simulink model "phase3_attitude_control"  (R2017b)
settings: Solver=VariableStepAuto  StartTime=0.0  StopTime=0.3  FixedStep=au  RelTol=1e-3
values from neighbouring files (symbols this model uses):
  c = 1.140*10^-7    (= 1.14e-07)    [Fcn_references_and_parameters.m]    (also in run_this_and_plot.m)
  Ix = 4.856*10^(-3)    (= 0.004856)    [Fcn_references_and_parameters.m]    (also in run_this_and_plot.m)
  Iy = 4.856*10^(-3)    (= 0.004856)    [Fcn_references_and_parameters.m]    (also in run_this_and_plot.m)
  Iz = 8.801*10^(-3)    (= 0.008801)    [Fcn_references_and_parameters.m]    (also in run_this_and_plot.m)
  k = 2.980*10^-6    (= 2.98e-06)    [Fcn_references_and_parameters.m]    (also in run_this_and_plot.m)
  l = 0.225    [Fcn_references_and_parameters.m]    (also in run_this_and_plot.m)
settings Model: Creator=Administrator  LastModifiedBy=chenjiasheng
settings CodeAppCC: StateflowObjectComments=on

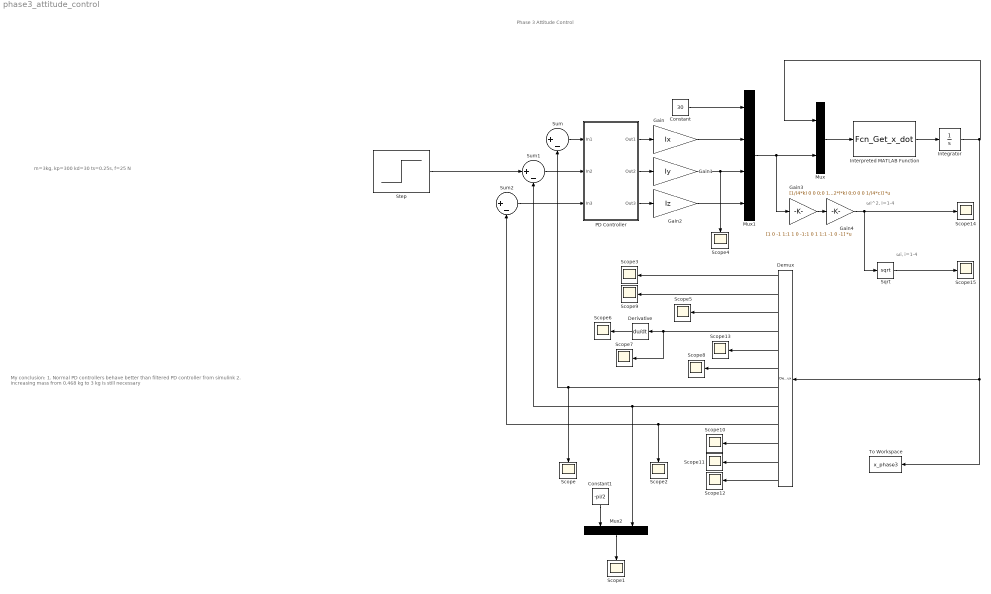
== system phase3_attitude_control ==
  note: My conclusion:
      | 1. Normal PD controllers behave better than filtered PD controller from simulink
      | 2. increasing mass from 0.468 kg to 3 kg is still necessary
  note: m=3kg, kp=300 kd=30 ts=0.25s, f=25 N
  note: Phase 3 Attitude Control
  note: ωi^2, i=1-4
  note: ωi, i=1-4
  Constant : Constant  Value=30
  Constant1 : Constant  Value=-pi/2
  Demux : Demux  Outputs=12
  Derivative : Derivative
  Gain : Gain  Gain=Ix
  Gain1 : Gain  Gain=Iy
  Gain2 : Gain  Gain=Iz
  Gain3 : Gain  Gain=[1/(4*k) 0 0 0;0 1/(2*l*k) 0 0;0 0 1/(2*l*k) 0;0 0 0 1/(4*c)]  Multiplication=Matrix(K*u) (u vector)
  Gain4 : Gain  Gain=[1 0 -1 1;1 1 0 -1;1 0 1 1;1 -1 0 -1]  Multiplication=Matrix(K*u) (u vector)
  Integrator : Integrator  InitialCondition=x_phase2(end,:)
  Interpreted MATLAB Function : MATLABFcn  MATLABFcn=Fcn_Get_x_dot
  Mux : Mux  Inputs=2
  Mux1 : Mux
  Mux2 : Mux  Inputs=2
  PD Controller : Subsystem
  Scope{,1..15} (16 alike) : Scope
  Sqrt : Sqrt  SaturateOnIntegerOverflow=on
  Step : Step  Time=0  After=-pi/2  SampleTime=0
  Sum : Sum  Inputs=|+-
  Sum1 : Sum  Inputs=|+-
  Sum2 : Sum  Inputs=|+-
  To Workspace : ToWorkspace  VariableName=x_phase3  SampleTime=0.01
  wires:
  Mux/1 -> Interpreted MATLAB Function/1
  Interpreted MATLAB Function/1 -> Integrator/1
  Integrator/1 -> To Workspace/1, Demux/1, Mux/1
  Mux1/1 -> Gain3/1, Mux/2
  Gain/1 -> Mux1/2
  Gain1/1 -> Scope4/1, Mux1/3
  Gain2/1 -> Mux1/4
  Demux/7 -> Scope/1, Sum/2
  Demux/8 -> Mux2/2, Sum1/2
  Demux/9 -> Scope2/1, Sum2/2
  Demux/3 -> Scope5/1
  Demux/4 -> Scope7/1, Derivative/1
  Demux/6 -> Scope8/1
  Derivative/1 -> Scope6/1
  Demux/1 -> Scope3/1
  Demux/2 -> Scope9/1
  Demux/10 -> Scope10/1
  Demux/11 -> Scope11/1
  Demux/12 -> Scope12/1
  Step/1 -> Sum1/1
  Demux/5 -> Scope13/1
  Mux2/1 -> Scope1/1
  Constant1/1 -> Mux2/1
  Gain3/1 -> Gain4/1
  Gain4/1 -> Scope14/1, Sqrt/1
  Constant/1 -> Mux1/1
  Sum/1 -> PD Controller/1(In1)
  PD Controller/1(Out1) -> Gain/1
  Sum1/1 -> PD Controller/2(In2)
  PD Controller/2(Out2) -> Gain1/1
  Sum2/1 -> PD Controller/3(In3)
  PD Controller/3(Out3) -> Gain2/1
  Sqrt/1 -> Scope15/1

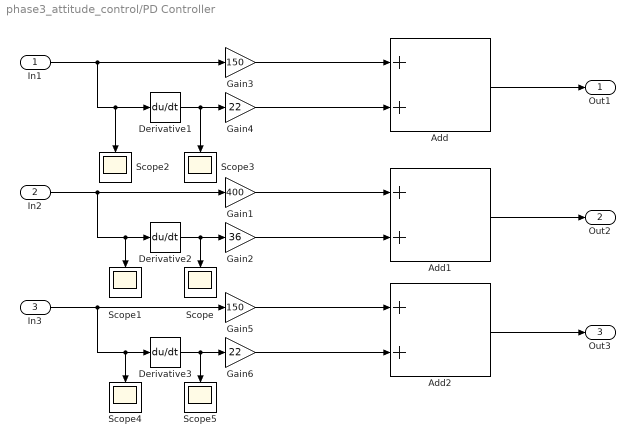
== system phase3_attitude_control/PD Controller ==
  In1 : Inport
  In2 : Inport  Port=2
  In3 : Inport  Port=3
  Add : Sum
  Add1 : Sum
  Add2 : Sum
  Derivative1 : Derivative
  Derivative2 : Derivative
  Derivative3 : Derivative
  Gain1 : Gain  Gain=400
  Gain2 : Gain  Gain=36
  Gain3 : Gain  Gain=150
  Gain4 : Gain  Gain=22
  Gain5 : Gain  Gain=150
  Gain6 : Gain  Gain=22
  Scope{,1..5} (6 alike) : Scope
  Out1 : Outport
  Out2 : Outport  Port=2
  Out3 : Outport  Port=3
  wires:
  In1/1 -> Scope2/1, Derivative1/1, Gain3/1
  Derivative1/1 -> Scope3/1, Gain4/1
  Add/1 -> Out1/1
  Add1/1 -> Out2/1
  Derivative2/1 -> Scope/1, Gain2/1
  Gain2/1 -> Add1/2
  In2/1 -> Gain1/1, Scope1/1, Derivative2/1
  Gain1/1 -> Add1/1
  In3/1 -> Scope4/1, Derivative3/1, Gain5/1
  Derivative3/1 -> Scope5/1, Gain6/1
  Add2/1 -> Out3/1
  Gain3/1 -> Add/1
  Gain5/1 -> Add2/1
  Gain6/1 -> Add2/2
  Gain4/1 -> Add/2
